simulink model "MRAC"  (Simulink 7.2)
settings: Solver=ode45  StartTime=0.0  StopTime=10.0  RelTol=1e-3
undefined symbols (not defined in the file): Am, B1, Bm, C, DZkx, DZtheta, flag_enable_adapt, flag_uad, Gamtheta, Gamx, in_error_thresh, in_t_timer, Kxhat0, Kxnom, Kxstar, Nrbf, P, Sig, Thetahat0, xm0
libraries: simulink x6
settings Model: Creator=E183308  LastModifiedBy=E183308

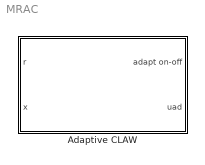
== system MRAC ==
  Adaptive CLAW : Subsystem

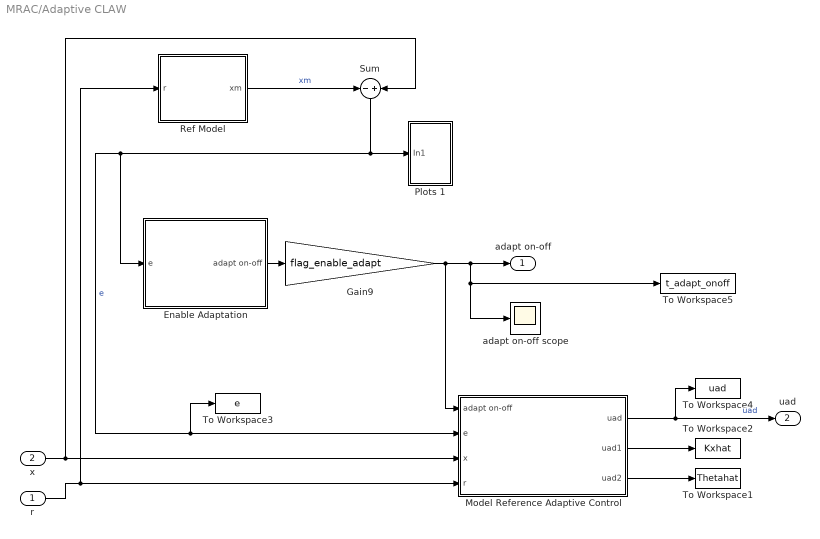
== system MRAC/Adaptive CLAW ==
  r : Inport
  x : Inport  Port=2
  Enable Adaptation : Subsystem
  Gain9 : Gain  Gain=flag_enable_adapt  ParameterDataType=sfix(16)  ParameterScaling=2^0  OutDataType=sfix(16)  OutScaling=2^0
  Model Reference Adaptive Control : Subsystem
  Plots 1 : Subsystem
  Ref Model : Subsystem
  Sum : Sum  Orientation=down  Inputs=-|+  OutDataType=sfix(16)  OutScaling=2^0
  To Workspace1 : ToWorkspace  VariableName=Thetahat  SampleTime=-1  SaveFormat=Array
  To Workspace2 : ToWorkspace  VariableName=Kxhat  SampleTime=-1  SaveFormat=Array
  To Workspace3 : ToWorkspace  VariableName=e  SampleTime=-1  SaveFormat=Array
  To Workspace4 : ToWorkspace  VariableName=uad  SampleTime=-1  SaveFormat=Array
  To Workspace5 : ToWorkspace  VariableName=t_adapt_onoff  SampleTime=-1  SaveFormat=Array
  adapt on-off scope : Scope
      settings: TimeRange=20  YMin=0  YMax=1  SaveName=ScopeData9
  adapt on-off : Outport
  uad : Outport  Port=2
  wires:
  Model Reference Adaptive Control/1(uad) -> uad/1, To Workspace4/1  "uad"
  Ref Model/1(xm) -> Sum/1  "xm"
  Sum/1 -> Plots 1/1(In1), Enable Adaptation/1(e), Model Reference Adaptive Control/2(e), To Workspace3/1  "e"
  x/1 -> Model Reference Adaptive Control/3(x), Sum/2
  r/1 -> Ref Model/1(r), Model Reference Adaptive Control/4(r)
  Enable Adaptation/1(adapt on-off) -> Gain9/1
  Model Reference Adaptive Control/2(uad1) -> To Workspace2/1
  Model Reference Adaptive Control/3(uad2) -> To Workspace1/1
  Gain9/1 -> Model Reference Adaptive Control/1(adapt on-off), adapt on-off/1, adapt on-off scope/1, To Workspace5/1

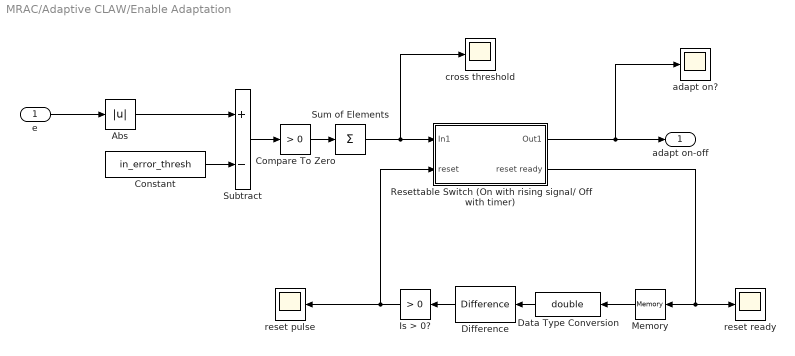
== system MRAC/Adaptive CLAW/Enable Adaptation ==
  e : Inport
  Abs : Abs  OutDataType=sfix(16)  OutScaling=2^0
  Compare To Zero : simulink/Logic and Bit Operations/Compare To Zero  SystemSampleTime=-1  relop=>  LogicOutDataTypeMode=uint8  ZeroCross=off
  Constant : Constant  Value=in_error_thresh  OutDataType=sfix(16)  OutScaling=2^0
  Data Type Conversion : DataTypeConversion  Orientation=left  OutDataTypeMode=double  OutDataType=sfix(16)  OutScaling=2^0  OutDataTypeStr=double
  Difference : simulink/Discrete/Difference  Orientation=left  SystemSampleTime=-1  ICPrevInput=1  OutMin=[]  OutMax=[]  OutDataType=sfix(16)  OutScaling=2^-10  DoSatur=off
  Is > 0? : simulink/Logic and Bit Operations/Compare To Zero  Orientation=left  SystemSampleTime=-1  relop=>  LogicOutDataTypeMode=boolean  ZeroCross=off
  Memory : Memory  Orientation=left  X0=1
  Resettable Switch (On with rising signal/ Off with timer) : Subsystem
  Subtract : Sum  Inputs=+-  OutDataType=sfix(16)  OutScaling=2^-10
  Sum of Elements : Sum  Inputs=+  OutDataType=sfix(16)  OutScaling=2^-10
  adapt on? : Scope
      settings: TimeRange=50  YMin=0  YMax=1  SaveName=ScopeData23
  cross threshold : Scope
      settings: TimeRange=50  YMin=0  YMax=1  SaveName=ScopeData22
  reset pulse : Scope
      settings: TimeRange=45  YMin=-1  YMax=1  SaveName=ScopeData20
  reset ready : Scope
      settings: TimeRange=20  YMin=0  YMax=1  SaveName=ScopeData21
  adapt on-off : Outport
  wires:
  Abs/1 -> Subtract/1
  Constant/1 -> Subtract/2
  Subtract/1 -> Compare To Zero/1
  e/1 -> Abs/1
  Compare To Zero/1 -> Sum of Elements/1
  Sum of Elements/1 -> Resettable Switch (On with rising signal/ Off with timer)/1(In1), cross threshold/1
  Resettable Switch (On with rising signal/ Off with timer)/1(Out1) -> adapt on-off/1, adapt on?/1
  Resettable Switch (On with rising signal/ Off with timer)/2(reset ready) -> reset ready/1, Memory/1
  Difference/1 -> Is > 0?/1
  Is > 0?/1 -> reset pulse/1, Resettable Switch (On with rising signal/ Off with timer)/2(reset)
  Data Type Conversion/1 -> Difference/1
  Memory/1 -> Data Type Conversion/1

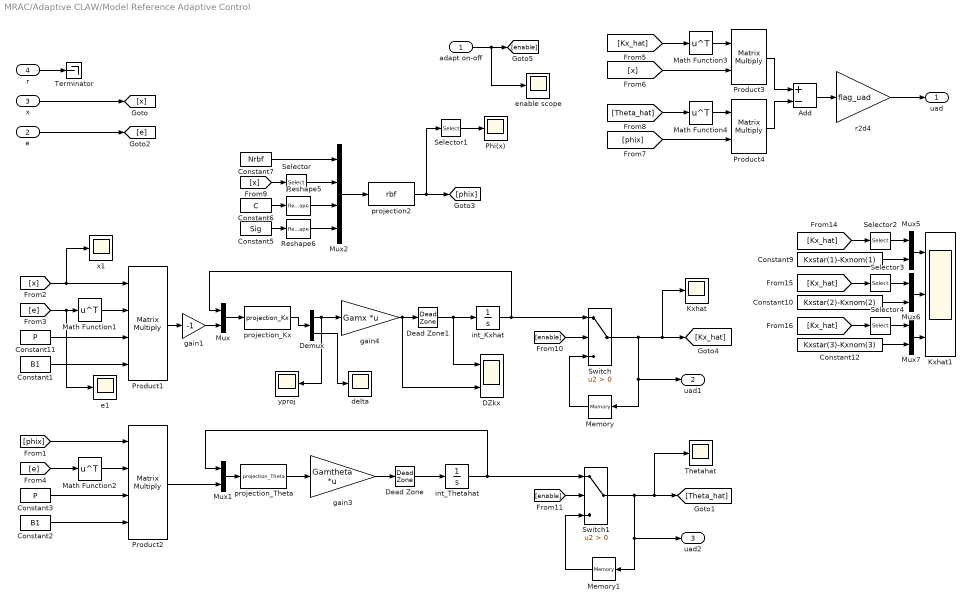
== system MRAC/Adaptive CLAW/Model Reference Adaptive Control ==
  adapt on-off : Inport  OutDataType=sfix(16)  OutScaling=2^0
  e : Inport  Port=2  OutDataType=sfix(16)  OutScaling=2^0
  x : Inport  Port=3  OutDataType=sfix(16)  OutScaling=2^0
  r : Inport  Port=4  OutDataType=sfix(16)  OutScaling=2^0
  Add : Sum  Inputs=+-  OutDataType=sfix(16)  OutScaling=2^-10
  Constant1 : Constant  Value=B1  OutDataType=sfix(16)  OutScaling=2^0
  Constant10 : Constant  Value=Kxstar(2)-Kxnom(2)  OutDataType=sfix(16)  OutScaling=2^0
  Constant11 : Constant  Value=P  OutDataType=sfix(16)  OutScaling=2^0
  Constant12 : Constant  Value=Kxstar(3)-Kxnom(3)  OutDataType=sfix(16)  OutScaling=2^0
  Constant2 : Constant  Value=B1  OutDataType=sfix(16)  OutScaling=2^0
  Constant3 : Constant  Value=P  OutDataType=sfix(16)  OutScaling=2^0
  Constant5 : Constant  Value=Sig  OutDataType=sfix(16)  OutScaling=2^0
  Constant6 : Constant  Value=C  OutDataType=sfix(16)  OutScaling=2^0
  Constant7 : Constant  Value=Nrbf  OutDataType=sfix(16)  OutScaling=2^0
  Constant9 : Constant  Value=Kxstar(1)-Kxnom(1)  OutDataType=sfix(16)  OutScaling=2^0
  DZkx : Scope  NumInputPorts=2
      settings: TimeRange=20  YMin=-150~-150  YMax=250~250  SaveName=ScopeData14
  Dead Zone : DeadZone  LowerValue=-DZtheta  UpperValue=DZtheta  SaturateOnIntegerOverflow=on
  Dead Zone1 : DeadZone  LowerValue=-DZkx  UpperValue=DZkx  SaturateOnIntegerOverflow=on
  Demux : Demux  Outputs=[3 3]
      settings: CopyFcn=set_param(gcbh,'ShowName','off','CopyFcn','')
  Kxhat : Scope
      settings: TimeRange=40  YMin=-0.05  YMax=0.15  SaveName=ScopeData4
  Kxhat1 : Scope  NumInputPorts=3
      settings: TimeRange=45  YMin=-50~-20~-50  YMax=150~140~200  SaveName=ScopeData13
  Math Function{1..4} (4 alike) : Math  Operator=transpose  OutDataType=sfix(16)  OutScaling=2^0  SaturateOnIntegerOverflow=on
  Memory : Memory  Orientation=left  X0=Kxhat0
  Memory1 : Memory  Orientation=left  X0=Thetahat0
  Mux : Mux  Inputs=2
  Mux1 : Mux  Inputs=2
  Mux2 : Mux
  Mux5 : Mux  Inputs=[1 1]
  Mux6 : Mux  Inputs=[1 1]
  Mux7 : Mux  Inputs=[1 1]
  Phi(x) : Scope
      settings: TimeRange=40  YMin=-0.05  YMax=0.9  SaveName=ScopeData12
  Product1 : Product  Inputs=4  Multiplication=Matrix(*)  OutDataType=sfix(16)  OutScaling=2^0  RndMeth=Zero
  Product2 : Product  Inputs=4  Multiplication=Matrix(*)  OutDataType=sfix(16)  OutScaling=2^0  RndMeth=Zero
  Product3 : Product  Multiplication=Matrix(*)  OutDataType=sfix(16)  OutScaling=2^0  RndMeth=Zero
  Product4 : Product  Multiplication=Matrix(*)  OutDataType=sfix(16)  OutScaling=2^0  RndMeth=Zero
  Reshape5 : Reshape  OutputDimensions=[1,Nrbf]
  Reshape6 : Reshape  OutputDimensions=[Nrbf,1]
  Selector : Selector  InputPortWidth=nx  IndexOptions=Index vector (dialog)  Indices=3  OutputSizes=1
  Selector1 : Selector  InputPortWidth=11  IndexOptions=Select all  Indices=5  OutputSizes=1
  Selector2 : Selector  InputPortWidth=3  IndexOptions=Index vector (dialog)  Indices=1  OutputSizes=1
  Selector3 : Selector  InputPortWidth=3  IndexOptions=Index vector (dialog)  Indices=2  OutputSizes=1
  Selector4 : Selector  InputPortWidth=3  IndexOptions=Index vector (dialog)  Indices=3  OutputSizes=1
  Switch : Switch  Criteria=u2 > Threshold
  Switch1 : Switch  Criteria=u2 > Threshold
  Terminator : Terminator
  Thetahat : Scope
      settings: TimeRange=40  YMin=-0.3  YMax=0.4  SaveName=ScopeData7
  delta : Scope
      settings: TimeRange=40  YMin=-0.05  YMax=0.9
  e1 : Scope
      settings: TimeRange=30  YMin=-400  YMax=500  SaveName=ScopeData19
  enable scope : Scope
      settings: TimeRange=40  YMin=-0.05  YMax=0.9  SaveName=ScopeData17
  gain1 : Gain  Gain=-1  ParameterDataType=sfix(16)  ParameterScaling=2^0  OutDataType=sfix(16)  OutScaling=2^0
  gain3 : Gain  Gain=Gamtheta  Multiplication=Matrix(K*u)  ParameterDataType=sfix(16)  ParameterScaling=2^0  OutDataType=sfix(16)  OutScaling=2^0
  gain4 : Gain  Gain=Gamx  Multiplication=Matrix(K*u)  ParameterDataType=sfix(16)  ParameterScaling=2^0  OutDataType=sfix(16)  OutScaling=2^0
  int_Kxhat : Integrator  InitialCondition=Kxhat0
  int_Thetahat : Integrator  InitialCondition=Thetahat0
  projection2 : MATLABFcn  MATLABFcn=rbf  OutputDimensions=[Nrbf,1]  Output1D=off
  projection_Kx : MATLABFcn  MATLABFcn=projection_Kx
  projection_Theta : MATLABFcn  MATLABFcn=projection_Theta
  r2d4 : Gain  Gain=flag_uad  ParameterDataType=sfix(16)  ParameterScaling=2^0  OutDataType=sfix(16)  OutScaling=2^0
  x1 : Scope
      settings: TimeRange=40  YMin=-0.1  YMax=0.15  SaveName=ScopeData18
  yproj : Scope
      settings: TimeRange=40  YMin=-0.05  YMax=0.9  SaveName=ScopeData2
  uad : Outport  OutDataType=sfix(16)  OutScaling=2^0  InitialOutput=0
  uad1 : Outport  Port=2  OutDataType=sfix(16)  OutScaling=2^0  InitialOutput=0
  uad2 : Outport  Port=3  OutDataType=sfix(16)  OutScaling=2^0  InitialOutput=0
  wires:
  r/1 -> Terminator/1
  e/1 -> [e]
  int_Kxhat/1 -> Mux/1, Switch/1
  [e] -> Math Function1/1, e1/1
  [Kx_hat] -> Math Function3/1
  Math Function3/1 -> Product3/1
  [x] -> Product3/2
  Product1/1 -> gain1/1
  [x] -> Product1/1, x1/1
  Math Function1/1 -> Product1/2
  Constant11/1 -> Product1/3
  Constant1/1 -> Product1/4
  x/1 -> [x]
  gain1/1 -> Mux/2
  Mux/1 -> projection_Kx/1
  int_Thetahat/1 -> Mux1/1, Switch1/1
  [e] -> Math Function2/1
  Product2/1 -> Mux1/2
  [phix] -> Product2/1
  Math Function2/1 -> Product2/2
  Constant3/1 -> Product2/3
  Constant2/1 -> Product2/4
  projection_Theta/1 -> gain3/1
  gain3/1 -> Dead Zone/1
  Mux1/1 -> projection_Theta/1
  [Theta_hat] -> Math Function4/1
  Math Function4/1 -> Product4/1
  [phix] -> Product4/2
  Product3/1 -> Add/1
  Product4/1 -> Add/2
  Add/1 -> r2d4/1
  Constant6/1 -> Reshape5/1
  Constant5/1 -> Reshape6/1
  Mux2/1 -> projection2/1
  projection2/1 -> [phix], Selector1/1
  Constant7/1 -> Mux2/1
  [x] -> Selector/1
  Reshape5/1 -> Mux2/3
  Reshape6/1 -> Mux2/4
  Selector/1 -> Mux2/2
  r2d4/1 -> uad/1
  Selector1/1 -> Phi(x)/1
  Dead Zone/1 -> int_Thetahat/1
  [Kx_hat] -> Selector2/1
  Selector2/1 -> Mux5/1
  Constant9/1 -> Mux5/2
  [Kx_hat] -> Selector3/1
  Selector3/1 -> Mux6/1
  Constant10/1 -> Mux6/2
  [Kx_hat] -> Selector4/1
  Selector4/1 -> Mux7/1
  Constant12/1 -> Mux7/2
  Mux5/1 -> Kxhat1/1
  Mux6/1 -> Kxhat1/2
  Mux7/1 -> Kxhat1/3
  Dead Zone1/1 -> DZkx/1, int_Kxhat/1
  gain4/1 -> Dead Zone1/1, DZkx/2
  projection_Kx/1 -> Demux/1
  Demux/1 -> gain4/1, yproj/1
  Demux/2 -> delta/1
  Switch1/1 -> [Theta_hat], Thetahat/1, uad2/1, Memory1/1
  [enable] -> Switch1/2
  Switch/1 -> [Kx_hat], Kxhat/1, uad1/1, Memory/1
  [enable] -> Switch/2
  adapt on-off/1 -> [enable], enable scope/1
  Memory1/1 -> Switch1/3
  Memory/1 -> Switch/3

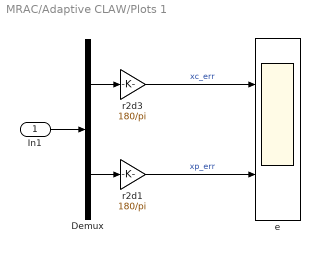
== system MRAC/Adaptive CLAW/Plots 1 ==
  In1 : Inport  OutDataType=sfix(16)  OutScaling=2^0
  Demux : Demux  Outputs=[1 2]
  e : Scope  NumInputPorts=2
      settings: TimeRange=60  YMin=-0.5~-2  YMax=2.5~2  SaveName=ScopeData6
  r2d1 : Gain  Gain=180/pi  ParameterDataType=sfix(16)  ParameterScaling=2^0  OutDataType=sfix(16)  OutScaling=2^0
  r2d3 : Gain  Gain=180/pi  ParameterDataType=sfix(16)  ParameterScaling=2^0  OutDataType=sfix(16)  OutScaling=2^0
  wires:
  Demux/1 -> r2d3/1
  r2d3/1 -> e/1  "xc_err"
  In1/1 -> Demux/1
  Demux/2 -> r2d1/1
  r2d1/1 -> e/2  "xp_err"

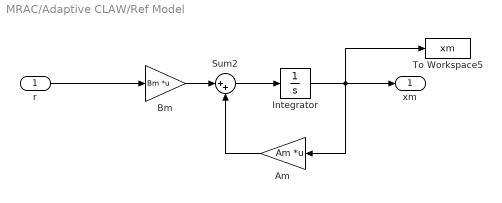
== system MRAC/Adaptive CLAW/Ref Model ==
  r : Inport  OutDataType=sfix(16)  OutScaling=2^0
  Am : Gain  Orientation=left  Gain=Am  Multiplication=Matrix(K*u)  ParameterDataType=sfix(16)  ParameterScaling=2^0  OutDataType=sfix(16)  OutScaling=2^0
  Bm : Gain  Gain=Bm  Multiplication=Matrix(K*u)  ParameterDataType=sfix(16)  ParameterScaling=2^0  OutDataType=sfix(16)  OutScaling=2^0
  Integrator : Integrator  InitialCondition=xm0
  Sum2 : Sum  Inputs=|++  OutDataType=sfix(16)  OutScaling=2^0
  To Workspace5 : ToWorkspace  VariableName=xm  SampleTime=-1  SaveFormat=Array
  xm : Outport  OutDataType=sfix(16)  OutScaling=2^0
  wires:
  r/1 -> Bm/1
  Integrator/1 -> Am/1, xm/1, To Workspace5/1
  Am/1 -> Sum2/2
  Sum2/1 -> Integrator/1
  Bm/1 -> Sum2/1

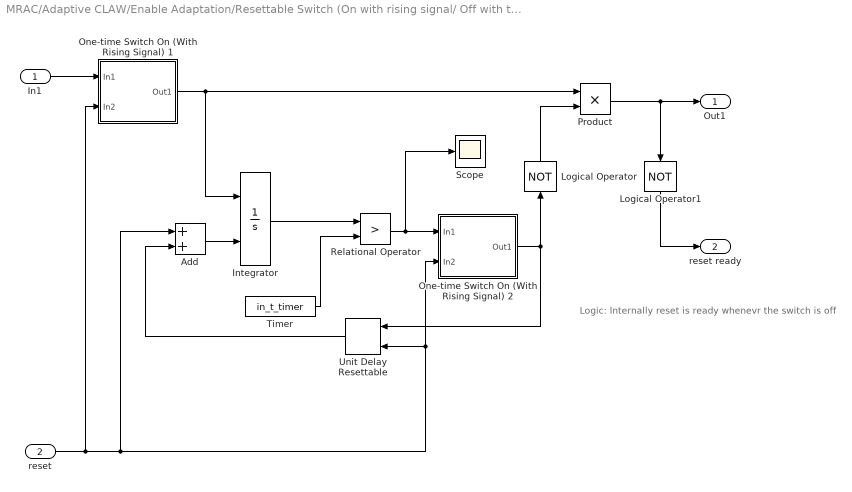
== system MRAC/Adaptive CLAW/Enable Adaptation/Resettable Switch (On with rising signal/ Off with timer) ==
  note: Logic: Internally reset
      | is ready whenevr
      | the switch is off
  In1 : Inport
  reset : Inport  Port=2
  Add : Sum  OutDataType=sfix(16)  OutScaling=2^-10
  Integrator : Integrator  ExternalReset=falling
  Logical Operator : Logic  Orientation=up  Operator=NOT  AllPortsSameDT=off  OutDataTypeMode=boolean  OutDataTypeStr=boolean
  Logical Operator1 : Logic  Orientation=down  Operator=NOT  AllPortsSameDT=off  OutDataTypeMode=boolean  OutDataTypeStr=boolean
  One-time Switch On (With Rising Signal) 1 : Subsystem
  One-time Switch On (With Rising Signal) 2 : Subsystem
  Product : Product  OutDataType=sfix(16)  OutScaling=2^0  RndMeth=Zero
  Relational Operator : RelationalOperator  Operator=>  LogicOutDataTypeMode=boolean  OutDataTypeStr=boolean
  Scope : Scope
      settings: TimeRange=1.5  YMin=0  YMax=2  SaveName=ScopeData8
  Timer : Constant  Value=in_t_timer  OutDataType=sfix(16)  OutScaling=2^0
  Unit Delay Resettable : simulink/Additional Math & Discrete/Additional Discrete/Unit Delay Resettable  Orientation=left  SystemSampleTime=-1  vinit=0.0  tsamp=-1
  Out1 : Outport
  reset ready : Outport  Port=2
  wires:
  Product/1 -> Out1/1, Logical Operator1/1
  In1/1 -> One-time Switch On (With Rising Signal) 1/1(In1)
  One-time Switch On (With Rising Signal) 2/1(Out1) -> Logical Operator/1, Unit Delay Resettable/1
  Timer/1 -> Relational Operator/2
  Relational Operator/1 -> One-time Switch On (With Rising Signal) 2/1(In1), Scope/1
  Integrator/1 -> Relational Operator/1
  One-time Switch On (With Rising Signal) 1/1(Out1) -> Integrator/1, Product/1
  reset/1 -> One-time Switch On (With Rising Signal) 1/2(In2), Unit Delay Resettable/2, One-time Switch On (With Rising Signal) 2/2(In2), Add/1
  Add/1 -> Integrator/2
  Unit Delay Resettable/1 -> Add/2
  Logical Operator/1 -> Product/2
  Logical Operator1/1 -> reset ready/1

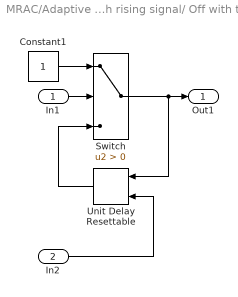
== system MRAC/Adaptive CLAW/Enable Adaptation/Resettable Switch (On with rising signal/ Off with timer)/One-time Switch On (With Rising Signal) 1 ==
  In1 : Inport
  In2 : Inport  Port=2
  Constant1 : Constant  OutDataType=sfix(16)  OutScaling=2^0
  Switch : Switch  Criteria=u2 > Threshold  OutDataType=sfix(16)  OutScaling=2^0
  Unit Delay Resettable : simulink/Additional Math & Discrete/Additional Discrete/Unit Delay Resettable  Orientation=left  SystemSampleTime=-1  vinit=0.0  tsamp=-1
  Out1 : Outport
  wires:
  In1/1 -> Switch/2
  Switch/1 -> Out1/1, Unit Delay Resettable/1
  Unit Delay Resettable/1 -> Switch/3
  Constant1/1 -> Switch/1
  In2/1 -> Unit Delay Resettable/2

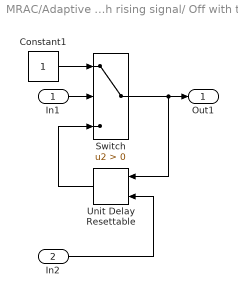
== system MRAC/Adaptive CLAW/Enable Adaptation/Resettable Switch (On with rising signal/ Off with timer)/One-time Switch On (With Rising Signal) 2 ==
  In1 : Inport
  In2 : Inport  Port=2
  Constant1 : Constant  OutDataType=sfix(16)  OutScaling=2^0
  Switch : Switch  Criteria=u2 > Threshold  OutDataType=sfix(16)  OutScaling=2^0
  Unit Delay Resettable : simulink/Additional Math & Discrete/Additional Discrete/Unit Delay Resettable  Orientation=left  SystemSampleTime=-1  vinit=0.0  tsamp=-1
  Out1 : Outport
  wires:
  In2/1 -> Unit Delay Resettable/2
  Constant1/1 -> Switch/1
  Unit Delay Resettable/1 -> Switch/3
  Switch/1 -> Unit Delay Resettable/1, Out1/1
  In1/1 -> Switch/2
